simulink model "chap8_5sim"  (Simulink 5.0)
settings: Solver=ode45  StartTime=0.0  StopTime=5  FixedStep=0.001  RelTol=1e-3
settings Model: LastModifiedBy=Administrator  ExtModeTrigMode=oneshot  ExtModeArmWhenConnect=off  LimitDataPoints=off  BooleanDataType=off

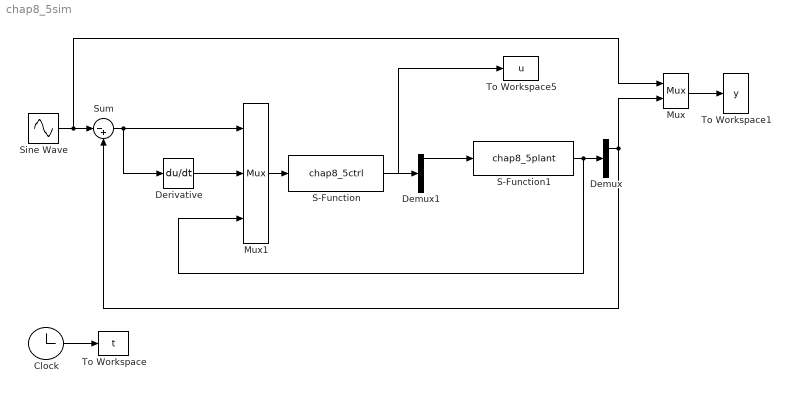
== system chap8_5sim ==
  Clock : Clock
  Demux : Demux  Outputs=2
  Demux1 : Demux
  Derivative : Derivative
  Mux : Mux  Inputs=2
  Mux1 : Mux  Inputs=3
  S-Function : S-Function  FunctionName=chap8_5ctrl
  S-Function1 : S-Function  FunctionName=chap8_5plant
  Sine Wave : Sin  Frequency=pi  SampleTime=0
  Sum : Sum  Inputs=|-+  SaturateOnIntegerOverflow=on
  To Workspace : ToWorkspace  VariableName=t  SampleTime=-1  SaveFormat=Array
  To Workspace1 : ToWorkspace  VariableName=y  SampleTime=-1  SaveFormat=Array
  To Workspace5 : ToWorkspace  VariableName=u  SampleTime=-1  SaveFormat=Array
  wires:
  Mux1/1 -> S-Function/1
  Mux/1 -> To Workspace1/1
  Demux/1 -> Mux/2, Sum/2
  S-Function1/1 -> Demux/1, Mux1/3
  Sine Wave/1 -> Sum/1, Mux/1
  Sum/1 -> Mux1/1, Derivative/1
  Derivative/1 -> Mux1/2
  S-Function/1 -> To Workspace5/1, Demux1/1
  Demux1/1 -> S-Function1/1
  Clock/1 -> To Workspace/1
